simulink model "pmc"  (Simulink 7.2)
settings: Solver=ode45  StartTime=0.0  StopTime=10.0  RelTol=1e-3
libraries: cdsEpicsOut x29, cdsFilt x23, cdsEpicsIn x12, cdsIPCx x10, dac x1, cdsParameters x1
(part 1 of 2)
settings Model: Creator=rolf  LastModifiedBy=rolf  ExtModeAutoUpdateStatusClock=off
settings OptimizationCC: InitFltsAndDblsToZero=on
settings DebuggingCC: SaveWithParameterizedLinksMsg=none  SignalResolutionControl=TryResolveAllWithWarning
settings GRTTargetCC: TargetFcnLib=ansi_tfl_tmw.mat

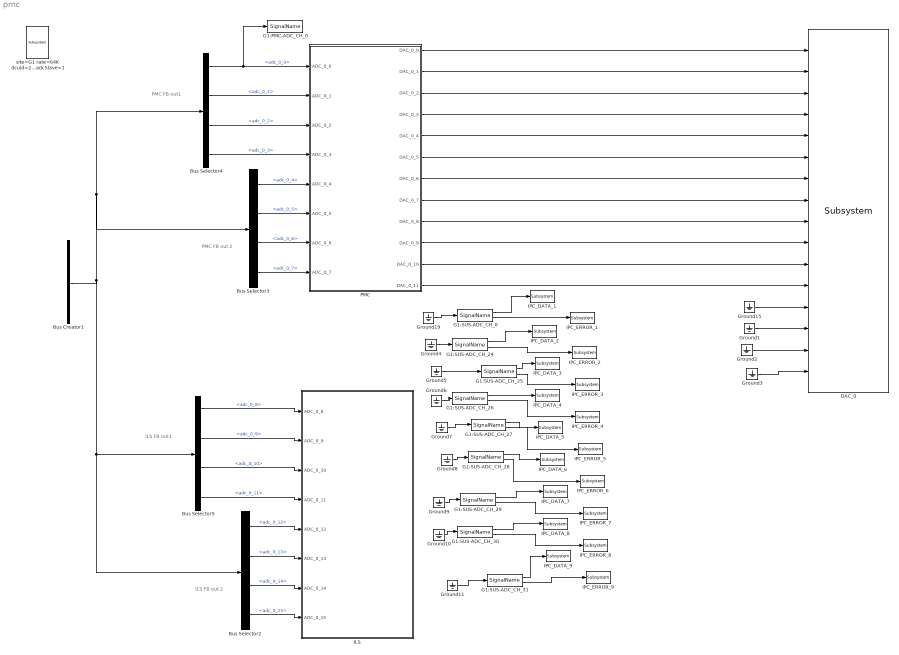
== system pmc ==
  note: PMC FB out 2
  note: PMC FB out1
  note: ILS FB out 2
  note: ILS FB out1
  Bus Creator1 : BusCreator  Tag=adc_1  Description=|  Inputs='adc_0_0','adc_0_1','adc_0_2','adc_0_3','adc_0_4','adc_0_5','adc_0_6','adc_0_7','adc_0_8','adc_0_9','adc_0_10','adc_0_11','adc_0_12','adc_0_13','adc_0_14','adc_0_15','adc_0_16','adc_0_17','adc_0_18','adc_0_19','adc_0_20','adc_0_21','adc_0_22','adc_0_23','adc_0_24','adc_0_25','adc_0_26','adc_0_27','adc_0_28','adc_0_29','adc_0_30','adc_0_31'
      | ADC1      
      | card_num=1
      settings: AttributesFormatString=%<Tag>
  Bus Selector2 : BusSelector  Description=ADC Selector  OutputSignals=adc_0_12,adc_0_13,adc_0_14,adc_0_15
      settings: AttributesFormatString=%<Description>
  Bus Selector3 : BusSelector  Description=ADC Selector  OutputSignals=adc_0_4,adc_0_5,adc_0_6,adc_0_7
      settings: AttributesFormatString=%<Description>
  Bus Selector4 : BusSelector  Description=ADC Selector  OutputSignals=adc_0_0,adc_0_1,adc_0_2,adc_0_3
      settings: AttributesFormatString=%<Description>
  Bus Selector5 : BusSelector  Description=ADC Selector  OutputSignals=adc_0_8,adc_0_9,adc_0_10,adc_0_11
      settings: AttributesFormatString=%<Description>
  DAC_0 : dac/Subsystem  Description=card_num=1  SystemSampleTime=-1
  G1:PMC-ADC_CH_0 : cdsIPCx/SignalName  Tag=cdsIPCx  Description=|  SystemSampleTime=-1
      | Inter-Process Communication via Shared memory, via Reflected
      | Memory network, or via PCI Express network.
      settings: AttributesFormatString=%<Tag>
  G1:SUS-ADC_CH_{0,24..31} (9 alike) : cdsIPCx/SignalName  Tag=cdsIPCx  Description=|  SystemSampleTime=-1
      | Inter-Process Communication via Shared memory, via Reflected
      | Memory network, or via PCI Express network.
      settings: AttributesFormatString=%<Tag>
  Ground{1..11,15,19} (13 alike) : Ground
  ILS : Subsystem
  IPC_DATA_1 : cdsEpicsOut/Subsystem  Tag=cdsEpicsOutput  Description=|  SystemSampleTime=-1
      | Purpose:                                          
      | Output a FE signal to an EPICS channel.           
      |                                                   
      | Operation:                                        
      | Takes input value and passes it to EPICS record.  
      |                                                   
      | Usage:                                            
      | Name the part with the desired EPICS rrecord name.
      settings: AttributesFormatString=%<Tag>
  IPC_DATA_2 : cdsEpicsOut/Subsystem  Tag=cdsEpicsOutput  Description=|  SystemSampleTime=-1
      | Purpose:                                          
      | Output a FE signal to an EPICS channel.           
      |                                                   
      | Operation:                                        
      | Takes input value and passes it to EPICS record.  
      |                                                   
      | Usage:                                            
      | Name the part with the desired EPICS rrecord name.
      settings: AttributesFormatString=%<Tag>
  IPC_DATA_3 : cdsEpicsOut/Subsystem  Tag=cdsEpicsOutput  Description=|  SystemSampleTime=-1
      | Purpose:                                          
      | Output a FE signal to an EPICS channel.           
      |                                                   
      | Operation:                                        
      | Takes input value and passes it to EPICS record.  
      |                                                   
      | Usage:                                            
      | Name the part with the desired EPICS rrecord name.
      settings: AttributesFormatString=%<Tag>
  IPC_DATA_4 : cdsEpicsOut/Subsystem  Tag=cdsEpicsOutput  Description=|  SystemSampleTime=-1
      | Purpose:                                          
      | Output a FE signal to an EPICS channel.           
      |                                                   
      | Operation:                                        
      | Takes input value and passes it to EPICS record.  
      |                                                   
      | Usage:                                            
      | Name the part with the desired EPICS rrecord name.
      settings: AttributesFormatString=%<Tag>
  IPC_DATA_5 : cdsEpicsOut/Subsystem  Tag=cdsEpicsOutput  Description=|  SystemSampleTime=-1
      | Purpose:                                          
      | Output a FE signal to an EPICS channel.           
      |                                                   
      | Operation:                                        
      | Takes input value and passes it to EPICS record.  
      |                                                   
      | Usage:                                            
      | Name the part with the desired EPICS rrecord name.
      settings: AttributesFormatString=%<Tag>
  IPC_DATA_6 : cdsEpicsOut/Subsystem  Tag=cdsEpicsOutput  Description=|  SystemSampleTime=-1
      | Purpose:                                          
      | Output a FE signal to an EPICS channel.           
      |                                                   
      | Operation:                                        
      | Takes input value and passes it to EPICS record.  
      |                                                   
      | Usage:                                            
      | Name the part with the desired EPICS rrecord name.
      settings: AttributesFormatString=%<Tag>
  IPC_DATA_7 : cdsEpicsOut/Subsystem  Tag=cdsEpicsOutput  Description=|  SystemSampleTime=-1
      | Purpose:                                          
      | Output a FE signal to an EPICS channel.           
      |                                                   
      | Operation:                                        
      | Takes input value and passes it to EPICS record.  
      |                                                   
      | Usage:                                            
      | Name the part with the desired EPICS rrecord name.
      settings: AttributesFormatString=%<Tag>
  IPC_DATA_8 : cdsEpicsOut/Subsystem  Tag=cdsEpicsOutput  Description=|  SystemSampleTime=-1
      | Purpose:                                          
      | Output a FE signal to an EPICS channel.           
      |                                                   
      | Operation:                                        
      | Takes input value and passes it to EPICS record.  
      |                                                   
      | Usage:                                            
      | Name the part with the desired EPICS rrecord name.
      settings: AttributesFormatString=%<Tag>
  IPC_DATA_9 : cdsEpicsOut/Subsystem  Tag=cdsEpicsOutput  Description=|  SystemSampleTime=-1
      | Purpose:                                          
      | Output a FE signal to an EPICS channel.           
      |                                                   
      | Operation:                                        
      | Takes input value and passes it to EPICS record.  
      |                                                   
      | Usage:                                            
      | Name the part with the desired EPICS rrecord name.
      settings: AttributesFormatString=%<Tag>
  IPC_ERROR_1 : cdsEpicsOut/Subsystem  Tag=cdsEpicsOutput  Description=|  SystemSampleTime=-1
      | Purpose:                                          
      | Output a FE signal to an EPICS channel.           
      |                                                   
      | Operation:                                        
      | Takes input value and passes it to EPICS record.  
      |                                                   
      | Usage:                                            
      | Name the part with the desired EPICS rrecord name.
      settings: AttributesFormatString=%<Tag>
  IPC_ERROR_2 : cdsEpicsOut/Subsystem  Tag=cdsEpicsOutput  Description=|  SystemSampleTime=-1
      | Purpose:                                          
      | Output a FE signal to an EPICS channel.           
      |                                                   
      | Operation:                                        
      | Takes input value and passes it to EPICS record.  
      |                                                   
      | Usage:                                            
      | Name the part with the desired EPICS rrecord name.
      settings: AttributesFormatString=%<Tag>
  IPC_ERROR_3 : cdsEpicsOut/Subsystem  Tag=cdsEpicsOutput  Description=|  SystemSampleTime=-1
      | Purpose:                                          
      | Output a FE signal to an EPICS channel.           
      |                                                   
      | Operation:                                        
      | Takes input value and passes it to EPICS record.  
      |                                                   
      | Usage:                                            
      | Name the part with the desired EPICS rrecord name.
      settings: AttributesFormatString=%<Tag>
  IPC_ERROR_4 : cdsEpicsOut/Subsystem  Tag=cdsEpicsOutput  Description=|  SystemSampleTime=-1
      | Purpose:                                          
      | Output a FE signal to an EPICS channel.           
      |                                                   
      | Operation:                                        
      | Takes input value and passes it to EPICS record.  
      |                                                   
      | Usage:                                            
      | Name the part with the desired EPICS rrecord name.
      settings: AttributesFormatString=%<Tag>
  IPC_ERROR_5 : cdsEpicsOut/Subsystem  Tag=cdsEpicsOutput  Description=|  SystemSampleTime=-1
      | Purpose:                                          
      | Output a FE signal to an EPICS channel.           
      |                                                   
      | Operation:                                        
      | Takes input value and passes it to EPICS record.  
      |                                                   
      | Usage:                                            
      | Name the part with the desired EPICS rrecord name.
      settings: AttributesFormatString=%<Tag>
  IPC_ERROR_6 : cdsEpicsOut/Subsystem  Tag=cdsEpicsOutput  Description=|  SystemSampleTime=-1
      | Purpose:                                          
      | Output a FE signal to an EPICS channel.           
      |                                                   
      | Operation:                                        
      | Takes input value and passes it to EPICS record.  
      |                                                   
      | Usage:                                            
      | Name the part with the desired EPICS rrecord name.
      settings: AttributesFormatString=%<Tag>
  IPC_ERROR_7 : cdsEpicsOut/Subsystem  Tag=cdsEpicsOutput  Description=|  SystemSampleTime=-1
      | Purpose:                                          
      | Output a FE signal to an EPICS channel.           
      |                                                   
      | Operation:                                        
      | Takes input value and passes it to EPICS record.  
      |                                                   
      | Usage:                                            
      | Name the part with the desired EPICS rrecord name.
      settings: AttributesFormatString=%<Tag>
  IPC_ERROR_8 : cdsEpicsOut/Subsystem  Tag=cdsEpicsOutput  Description=|  SystemSampleTime=-1
      | Purpose:                                          
      | Output a FE signal to an EPICS channel.           
      |                                                   
      | Operation:                                        
      | Takes input value and passes it to EPICS record.  
      |                                                   
      | Usage:                                            
      | Name the part with the desired EPICS rrecord name.
      settings: AttributesFormatString=%<Tag>
  IPC_ERROR_9 : cdsEpicsOut/Subsystem  Tag=cdsEpicsOutput  Description=|  SystemSampleTime=-1
      | Purpose:                                          
      | Output a FE signal to an EPICS channel.           
      |                                                   
      | Operation:                                        
      | Takes input value and passes it to EPICS record.  
      |                                                   
      | Usage:                                            
      | Name the part with the desired EPICS rrecord name.
      settings: AttributesFormatString=%<Tag>
  PMC : Subsystem
  site=G1 rate=64K dcuid=21 shmem_daq=1 gds_node_id=5 specific_cpu=5 adcSlave=1 : cdsParameters/Subsystem  Tag=cdsParameters  SystemSampleTime=-1
      settings: AttributesFormatString=%<Tag>
  wires:
  Bus Selector4/2 -> PMC/2(ADC_0_1)  "<adc_0_1>"
  Bus Selector3/2 -> PMC/6(ADC_0_5)  "<adc_0_5>"
  Bus Selector3/1 -> PMC/5(ADC_0_4)  "<adc_0_4>"
  Bus Selector4/3 -> PMC/3(ADC_0_2)  "<adc_0_2>"
  Bus Selector4/1 -> PMC/1(ADC_0_0), G1:PMC-ADC_CH_0/1  "<adc_0_0>"
  Bus Creator1/1 -> Bus Selector4/1, Bus Selector3/1, Bus Selector5/1, Bus Selector2/1
  Bus Selector4/4 -> PMC/4(ADC_0_3)  "<adc_0_3>"
  Bus Selector3/3 -> PMC/7(ADC_0_6)  "<adc_0_6>"
  Bus Selector3/4 -> PMC/8(ADC_0_7)  "<adc_0_7>"
  Bus Selector5/2 -> ILS/2(ADC_0_9)  "<adc_0_9>"
  Bus Selector2/2 -> ILS/6(ADC_0_13)  "<adc_0_13>"
  Bus Selector2/1 -> ILS/5(ADC_0_12)  "<adc_0_12>"
  Bus Selector5/3 -> ILS/3(ADC_0_10)  "<adc_0_10>"
  Bus Selector5/1 -> ILS/1(ADC_0_8)  "<adc_0_8>"
  Bus Selector5/4 -> ILS/4(ADC_0_11)  "<adc_0_11>"
  Bus Selector2/3 -> ILS/7(ADC_0_14)  "<adc_0_14>"
  Bus Selector2/4 -> ILS/8(ADC_0_15)  "<adc_0_15>"
  PMC/1(DAC_0_0) -> DAC_0/1
  PMC/2(DAC_0_1) -> DAC_0/2
  PMC/3(DAC_0_2) -> DAC_0/3
  PMC/4(DAC_0_3) -> DAC_0/4
  PMC/5(DAC_0_4) -> DAC_0/5
  PMC/6(DAC_0_5) -> DAC_0/6
  PMC/7(DAC_0_6) -> DAC_0/7
  PMC/8(DAC_0_7) -> DAC_0/8
  PMC/9(DAC_0_8) -> DAC_0/9
  PMC/10(DAC_0_9) -> DAC_0/10
  PMC/11(DAC_0_10) -> DAC_0/11
  PMC/12(DAC_0_11) -> DAC_0/12
  Ground15/1 -> DAC_0/13
  Ground1/1 -> DAC_0/14
  Ground2/1 -> DAC_0/15
  Ground3/1 -> DAC_0/16
  G1:SUS-ADC_CH_0/1 -> IPC_DATA_1/1
  G1:SUS-ADC_CH_0/2 -> IPC_ERROR_1/1
  G1:SUS-ADC_CH_31/1 -> IPC_DATA_9/1
  G1:SUS-ADC_CH_31/2 -> IPC_ERROR_9/1
  G1:SUS-ADC_CH_30/1 -> IPC_DATA_8/1
  G1:SUS-ADC_CH_30/2 -> IPC_ERROR_8/1
  G1:SUS-ADC_CH_29/1 -> IPC_DATA_7/1
  G1:SUS-ADC_CH_29/2 -> IPC_ERROR_7/1
  G1:SUS-ADC_CH_28/1 -> IPC_DATA_6/1
  G1:SUS-ADC_CH_28/2 -> IPC_ERROR_6/1
  G1:SUS-ADC_CH_27/1 -> IPC_DATA_5/1
  G1:SUS-ADC_CH_27/2 -> IPC_ERROR_5/1
  G1:SUS-ADC_CH_26/2 -> IPC_ERROR_4/1
  G1:SUS-ADC_CH_26/1 -> IPC_DATA_4/1
  G1:SUS-ADC_CH_25/1 -> IPC_DATA_3/1
  G1:SUS-ADC_CH_25/2 -> IPC_ERROR_3/1
  G1:SUS-ADC_CH_24/1 -> IPC_DATA_2/1
  G1:SUS-ADC_CH_24/2 -> IPC_ERROR_2/1
  Ground11/1 -> G1:SUS-ADC_CH_31/1
  Ground10/1 -> G1:SUS-ADC_CH_30/1
  Ground9/1 -> G1:SUS-ADC_CH_29/1
  Ground8/1 -> G1:SUS-ADC_CH_28/1
  Ground7/1 -> G1:SUS-ADC_CH_27/1
  Ground6/1 -> G1:SUS-ADC_CH_26/1
  Ground5/1 -> G1:SUS-ADC_CH_25/1
  Ground4/1 -> G1:SUS-ADC_CH_24/1
  Ground19/1 -> G1:SUS-ADC_CH_0/1

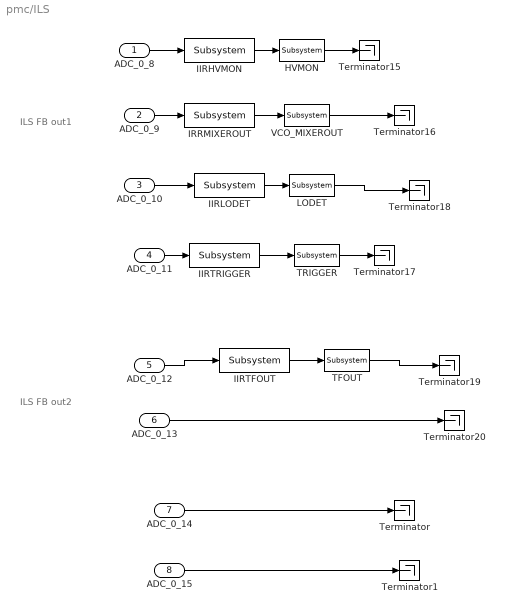
== system pmc/ILS ==
  note: ILS FB out1
  note: ILS FB out2
  ADC_0_8 : Inport  OutDataType=sfix(16)  OutScaling=2^0
  ADC_0_9 : Inport  Port=2  OutDataType=sfix(16)  OutScaling=2^0
  ADC_0_10 : Inport  Port=3  OutDataType=sfix(16)  OutScaling=2^0
  ADC_0_11 : Inport  Port=4  OutDataType=sfix(16)  OutScaling=2^0
  ADC_0_12 : Inport  Port=5  OutDataType=sfix(16)  OutScaling=2^0
  ADC_0_13 : Inport  Port=6  OutDataType=sfix(16)  OutScaling=2^0
  ADC_0_14 : Inport  Port=7  OutDataType=sfix(16)  OutScaling=2^0
  ADC_0_15 : Inport  Port=8  OutDataType=sfix(16)  OutScaling=2^0
  HVMON : cdsEpicsOut/Subsystem  Tag=cdsEpicsOutput  Description=|  SystemSampleTime=-1
      | Purpose:                                          
      | Output a FE signal to an EPICS channel.           
      |                                                   
      | Operation:                                        
      | Takes input value and passes it to EPICS record.  
      |                                                   
      | Usage:                                            
      | Name the part with the desired EPICS rrecord name.
      settings: AttributesFormatString=%<Tag>
  IIRHVMON : cdsFilt/Subsystem  Tag=cdsFilt  Description=|  SystemSampleTime=-1
      | Purpose:                                                                                                                                                                                                                                  
      | Standard CDS IIR filter module.                                                                                                                                                                                                           
      |                                                                                                                                                                                                                                           
      | Operation:                                                                                                                                                                                                                                
      | Consists of 10 second order section IIR filters, plus a ramped gain stage. In FE code, also provides pre-defined test points and excitation channel inputs. The filter coefficients are defined in the LIGO system using the 'foton' tool.
      |                                                                                                                                                                                                                                           
      | Usage:                                                                                                                                                                                                                                    
      | Name the part with the desired filter module name.
      settings: AttributesFormatString=%<Tag>
  IIRLODET : cdsFilt/Subsystem  Tag=cdsFilt  Description=|  SystemSampleTime=-1
      | Purpose:                                                                                                                                                                                                                                  
      | Standard CDS IIR filter module.                                                                                                                                                                                                           
      |                                                                                                                                                                                                                                           
      | Operation:                                                                                                                                                                                                                                
      | Consists of 10 second order section IIR filters, plus a ramped gain stage. In FE code, also provides pre-defined test points and excitation channel inputs. The filter coefficients are defined in the LIGO system using the 'foton' tool.
      |                                                                                                                                                                                                                                           
      | Usage:                                                                                                                                                                                                                                    
      | Name the part with the desired filter module name.
      settings: AttributesFormatString=%<Tag>
  IIRTFOUT : cdsFilt/Subsystem  Tag=cdsFilt  Description=|  SystemSampleTime=-1
      | Purpose:                                                                                                                                                                                                                                  
      | Standard CDS IIR filter module.                                                                                                                                                                                                           
      |                                                                                                                                                                                                                                           
      | Operation:                                                                                                                                                                                                                                
      | Consists of 10 second order section IIR filters, plus a ramped gain stage. In FE code, also provides pre-defined test points and excitation channel inputs. The filter coefficients are defined in the LIGO system using the 'foton' tool.
      |                                                                                                                                                                                                                                           
      | Usage:                                                                                                                                                                                                                                    
      | Name the part with the desired filter module name.
      settings: AttributesFormatString=%<Tag>
  IIRTRIGGER : cdsFilt/Subsystem  Tag=cdsFilt  Description=|  SystemSampleTime=-1
      | Purpose:                                                                                                                                                                                                                                  
      | Standard CDS IIR filter module.                                                                                                                                                                                                           
      |                                                                                                                                                                                                                                           
      | Operation:                                                                                                                                                                                                                                
      | Consists of 10 second order section IIR filters, plus a ramped gain stage. In FE code, also provides pre-defined test points and excitation channel inputs. The filter coefficients are defined in the LIGO system using the 'foton' tool.
      |                                                                                                                                                                                                                                           
      | Usage:                                                                                                                                                                                                                                    
      | Name the part with the desired filter module name.
      settings: AttributesFormatString=%<Tag>
  IRRMIXEROUT : cdsFilt/Subsystem  Tag=cdsFilt  Description=|  SystemSampleTime=-1
      | Purpose:                                                                                                                                                                                                                                  
      | Standard CDS IIR filter module.                                                                                                                                                                                                           
      |                                                                                                                                                                                                                                           
      | Operation:                                                                                                                                                                                                                                
      | Consists of 10 second order section IIR filters, plus a ramped gain stage. In FE code, also provides pre-defined test points and excitation channel inputs. The filter coefficients are defined in the LIGO system using the 'foton' tool.
      |                                                                                                                                                                                                                                           
      | Usage:                                                                                                                                                                                                                                    
      | Name the part with the desired filter module name.
      settings: AttributesFormatString=%<Tag>
  LODET : cdsEpicsOut/Subsystem  Tag=cdsEpicsOutput  Description=|  SystemSampleTime=-1
      | Purpose:                                          
      | Output a FE signal to an EPICS channel.           
      |                                                   
      | Operation:                                        
      | Takes input value and passes it to EPICS record.  
      |                                                   
      | Usage:                                            
      | Name the part with the desired EPICS rrecord name.
      settings: AttributesFormatString=%<Tag>
  TFOUT : cdsEpicsOut/Subsystem  Tag=cdsEpicsOutput  Description=|  SystemSampleTime=-1
      | Purpose:                                          
      | Output a FE signal to an EPICS channel.           
      |                                                   
      | Operation:                                        
      | Takes input value and passes it to EPICS record.  
      |                                                   
      | Usage:                                            
      | Name the part with the desired EPICS rrecord name.
      settings: AttributesFormatString=%<Tag>
  TRIGGER : cdsEpicsOut/Subsystem  Tag=cdsEpicsOutput  Description=|  SystemSampleTime=-1
      | Purpose:                                          
      | Output a FE signal to an EPICS channel.           
      |                                                   
      | Operation:                                        
      | Takes input value and passes it to EPICS record.  
      |                                                   
      | Usage:                                            
      | Name the part with the desired EPICS rrecord name.
      settings: AttributesFormatString=%<Tag>
  Terminator{,1,15..20} (8 alike) : Terminator
  VCO_MIXEROUT : cdsEpicsOut/Subsystem  Tag=cdsEpicsOutput  Description=|  SystemSampleTime=-1
      | Purpose:                                          
      | Output a FE signal to an EPICS channel.           
      |                                                   
      | Operation:                                        
      | Takes input value and passes it to EPICS record.  
      |                                                   
      | Usage:                                            
      | Name the part with the desired EPICS rrecord name.
      settings: AttributesFormatString=%<Tag>
  wires:
  HVMON/1 -> Terminator15/1
  IIRHVMON/1 -> HVMON/1
  TRIGGER/1 -> Terminator17/1
  IIRTRIGGER/1 -> TRIGGER/1
  ADC_0_8/1 -> IIRHVMON/1
  ADC_0_11/1 -> IIRTRIGGER/1
  ADC_0_9/1 -> IRRMIXEROUT/1
  ADC_0_10/1 -> IIRLODET/1
  IRRMIXEROUT/1 -> VCO_MIXEROUT/1
  VCO_MIXEROUT/1 -> Terminator16/1
  IIRLODET/1 -> LODET/1
  LODET/1 -> Terminator18/1
  IIRTFOUT/1 -> TFOUT/1
  ADC_0_12/1 -> IIRTFOUT/1
  TFOUT/1 -> Terminator19/1
  ADC_0_14/1 -> Terminator/1
  ADC_0_15/1 -> Terminator1/1
  ADC_0_13/1 -> Terminator20/1
